simulink model "Quadrotor_Model_CP232"  (R2020a)
settings: Solver=ode3  StartTime=0.0  StopTime=Tf  FixedStep=0.01  RelTol=1e-3  EnableMultiTasking=on
InitFcn:
  | %g = 9.81; % gravity constant m/s^2
  | %m = 0.468; % mass of helicopter kg
  | %l = 0.225; % distance between a rotor and the center of quadcopter (m)
  | %k = 2.98e-6; % lift constant
  | %b = 1.14e-7; % drag constant
  | %I_M = 3.357e-5; % rotational moment of inertia kg.m^2
  | % drag force coefficents
  | %A_x = 0.25; % kg/s
  | %A_y = 0.25;
  | %A_z = 0.25;
  | % inertia matrix
  | %I_xx = 4.856e-3; %kgm^2
  | %I_yy = 4.856e-3;
  | %I_zz = 8.801e-3;
values from neighbouring files (symbols this model uses):
  Fxg = 0.5*scale2    (= 0)    [main_no_wind.m]    (also in main_with_wind.m = 0.005)
  Fyg = 0.5*scale2    (= 0)    [main_no_wind.m]    (also in main_with_wind.m = 0.005)
  g = 9.8    [main_no_wind.m]    (also in main_with_wind.m)
  I = diag([2.3951 2.3951 3.2347])*1e-5    [main_no_wind.m]    (also in main_with_wind.m)
  I_xx = I(1,1)    [main_no_wind.m]    (also in main_with_wind.m)
  I_yy = I(2,2)    [main_no_wind.m]    (also in main_with_wind.m)
  I_zz = I(3,3)    [main_no_wind.m]    (also in main_with_wind.m)
  Kd_eta = [40; 50; 50]    [main_no_wind.m]    (also in main_with_wind.m = [200; 200; 10])
  Kd_zeta = [3; 100; 5]    [main_no_wind.m]    (also in main_with_wind.m = [10; 100; 5])
  kf = 0.005022    [main_no_wind.m]    (also in main_with_wind.m)
  Ki_eta = [0; 0; 0]    [main_no_wind.m]    (also in main_with_wind.m)
  Ki_zeta = [0; 0; 0]    [main_no_wind.m]    (also in main_with_wind.m = [10; 0; 0])
  km = 1.858e-5    (= 1.858e-05)    [main_no_wind.m]    (also in main_with_wind.m)
  Kp_eta = [20; 50; 50]    [main_no_wind.m]    (also in main_with_wind.m = [100; 100; 10])
  Kp_zeta = [2; 1; 1]    [main_no_wind.m]    (also in main_with_wind.m = [50; 50; 10])
  L = 0.032    [main_no_wind.m]    (also in main_with_wind.m)
  m = 0.034    [main_no_wind.m]    (also in main_with_wind.m)
  MMA = [0 kf*L 0 -kf*L;         -kf*L 0 kf*L 0;         km -km km -km]    [main_no_wind.m]    (also in main_with_wind.m)
  scale = 0    [main_no_wind.m]    (also in main_with_wind.m = 0.0001)
  shape = 0    [main_no_wind.m]    (also in main_with_wind.m)
  x_0 = 1    [main_no_wind.m]    (also in main_with_wind.m)
  y_0 = 0    [main_no_wind.m]    (also in main_with_wind.m)
  z_0 = 0    [main_no_wind.m]    (also in main_with_wind.m)
libraries: dspinverses x1
settings Model: Creator=Hamed  LastModifiedBy=Ratnangshu
settings DataIOCC: ReturnWorkspaceOutputs=off
settings OptimizationCC: LifeSpan=inf
settings DebuggingCC: SFUnexpectedBacktrackingDiag=warning  SFNoUnconditionalDefaultTransitionDiag=warning  SFExecutionAtInitializationDiag=none  ArithmeticOperatorsInVariantConditions=warning
settings HardwareCC: ProdBitPerSizeT=32  ProdBitPerPtrDiffT=32  ProdWordSize=32  ProdHWDeviceType=Specified
settings SFSimCC: SimUseLocalCustomCode=off  CustomCodeUndefinedFunction=UseInterfaceOnly
settings RTWCC: RTWUseLocalCustomCode=off
settings CodeAppCC: StateflowObjectComments=on
settings GRTTargetCC: TargetLangStandard=C89/C90 (ANSI)
settings ConfigComp: CovMetricSettings=dw  CovHtmlReporting=on  CovSaveCumulativeToWorkspaceVar=on  CovSaveSingleToWorkspaceVar=on  CovExternalEMLEnable=off

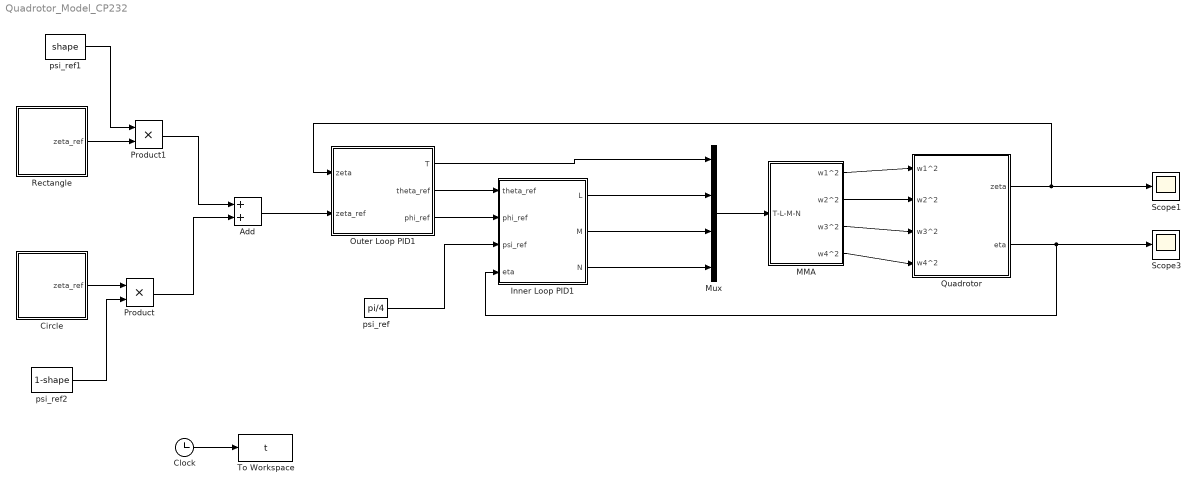
== system Quadrotor_Model_CP232 ==
  Add : Sum
  Circle : Subsystem
  Clock : Clock
  Inner Loop PID1 : Subsystem
  MMA : Subsystem
  Mux : Mux
  Outer Loop PID1 : Subsystem
  Product : Product
  Product1 : Product
  Quadrotor : Subsystem
  Rectangle : Subsystem
  Scope1 : Scope
  Scope3 : Scope
  To Workspace : ToWorkspace  VariableName=t  SampleTime=-1
  psi_ref : Constant  Value=pi/4
  psi_ref1 : Constant  Value=shape
  psi_ref2 : Constant  Value=1-shape
  wires:
  Mux/1 -> MMA/1(T-L-M-N)
  Inner Loop PID1/1(L) -> Mux/2
  Outer Loop PID1/2(theta_ref) -> Inner Loop PID1/1(theta_ref)
  Outer Loop PID1/3(phi_ref) -> Inner Loop PID1/2(phi_ref)
  psi_ref/1 -> Inner Loop PID1/3(psi_ref)
  Outer Loop PID1/1(T) -> Mux/1
  Inner Loop PID1/2(M) -> Mux/3
  Inner Loop PID1/3(N) -> Mux/4
  Quadrotor/1(zeta) -> Outer Loop PID1/1(zeta), Scope1/1
  Quadrotor/2(eta) -> Inner Loop PID1/4(eta), Scope3/1
  MMA/1(w1^2) -> Quadrotor/1(w1^2)
  MMA/2(w2^2) -> Quadrotor/2(w2^2)
  MMA/3(w3^2) -> Quadrotor/3(w3^2)
  MMA/4(w4^2) -> Quadrotor/4(w4^2)
  Add/1 -> Outer Loop PID1/2(zeta_ref)
  Rectangle/1(zeta_ref) -> Product1/2
  Circle/1(zeta_ref) -> Product/1
  Product/1 -> Add/2
  Product1/1 -> Add/1
  psi_ref1/1 -> Product1/1
  psi_ref2/1 -> Product/2
  Clock/1 -> To Workspace/1

== system Quadrotor_Model_CP232/Circle ==
  Clock : Clock
  MATLAB Function : MATLAB Function  TreatAsAtomicUnit=on
  MATLAB Function1 : MATLAB Function  TreatAsAtomicUnit=on
  MATLAB Function2 : MATLAB Function  TreatAsAtomicUnit=on
  Mux : Mux  Inputs=3
  zeta_ref : Outport
  wires:
  Clock/1 -> MATLAB Function2/1(t), MATLAB Function1/1(t), MATLAB Function/1(t)
  MATLAB Function/1(y_ref) -> Mux/2
  MATLAB Function1/1(x_ref) -> Mux/1
  MATLAB Function2/1(z_ref) -> Mux/3
  Mux/1 -> zeta_ref/1

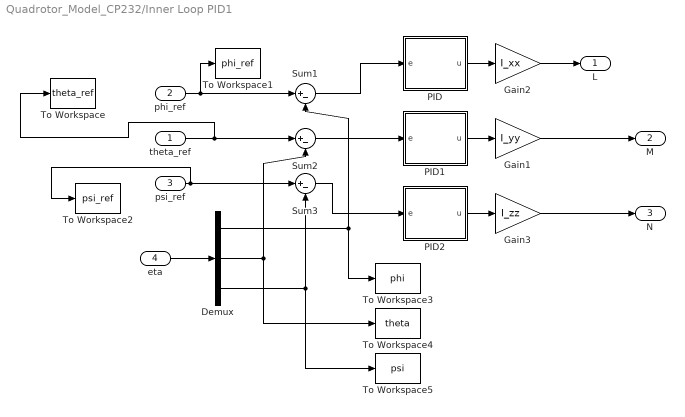
== system Quadrotor_Model_CP232/Inner Loop PID1 ==
  theta_ref : Inport
  phi_ref : Inport  Port=2
  psi_ref : Inport  Port=3
  eta : Inport  Port=4
  Demux : Demux  Outputs=3
  Gain1 : Gain  Gain=I_yy
  Gain2 : Gain  Gain=I_xx
  Gain3 : Gain  Gain=I_zz
  PID : Subsystem
  PID1 : Subsystem
  PID2 : Subsystem
  Sum1 : Sum  Inputs=|+-
  Sum2 : Sum  Inputs=|+-
  Sum3 : Sum  Inputs=|+-
  To Workspace : ToWorkspace  VariableName=theta_ref  SampleTime=-1
  To Workspace1 : ToWorkspace  VariableName=phi_ref  SampleTime=-1
  To Workspace2 : ToWorkspace  VariableName=psi_ref  SampleTime=-1
  To Workspace3 : ToWorkspace  VariableName=phi  SampleTime=-1
  To Workspace4 : ToWorkspace  VariableName=theta  SampleTime=-1
  To Workspace5 : ToWorkspace  VariableName=psi  SampleTime=-1
  L : Outport
  M : Outport  Port=2
  N : Outport  Port=3
  wires:
  PID2/1(u) -> Gain3/1
  PID1/1(u) -> Gain1/1
  PID/1(u) -> Gain2/1
  Gain3/1 -> N/1
  Gain1/1 -> M/1
  Gain2/1 -> L/1
  Demux/2 -> Sum2/2, To Workspace4/1
  Sum2/1 -> PID1/1(e)
  Demux/3 -> Sum3/2, To Workspace5/1
  Sum3/1 -> PID2/1(e)
  Sum1/1 -> PID/1(e)
  theta_ref/1 -> Sum2/1, To Workspace/1
  Demux/1 -> Sum1/2, To Workspace3/1
  phi_ref/1 -> Sum1/1, To Workspace1/1
  psi_ref/1 -> Sum3/1, To Workspace2/1
  eta/1 -> Demux/1

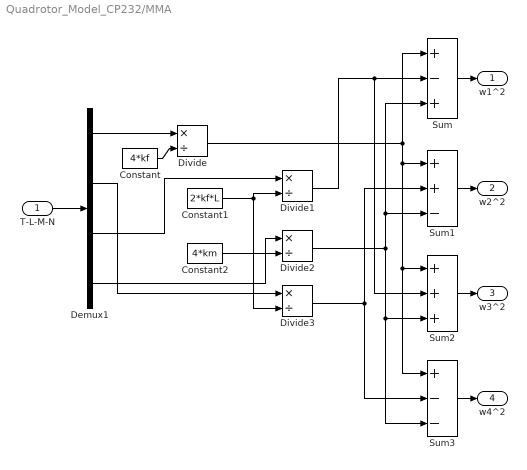
== system Quadrotor_Model_CP232/MMA ==
  T-L-M-N : Inport
  Constant : Constant  Value=4*kf
  Constant1 : Constant  Value=2*kf*L
  Constant2 : Constant  Value=4*km
  Demux1 : Demux
  Divide{,1..3} (4 alike) : Product  Inputs=*/
  Sum : Sum  Inputs=+-+
  Sum1 : Sum  Inputs=++-
  Sum2 : Sum  Inputs=+++
  Sum3 : Sum  Inputs=+--
  w1^2 : Outport
  w2^2 : Outport  Port=2
  w3^2 : Outport  Port=3
  w4^2 : Outport  Port=4
  wires:
  Sum1/1 -> w2^2/1
  T-L-M-N/1 -> Demux1/1
  Sum3/1 -> w4^2/1
  Sum/1 -> w1^2/1
  Demux1/2 -> Divide3/1
  Divide3/1 -> Sum1/2, Sum3/2
  Sum2/1 -> w3^2/1
  Constant/1 -> Divide/2
  Constant2/1 -> Divide2/2
  Demux1/1 -> Divide/1
  Demux1/3 -> Divide1/1
  Demux1/4 -> Divide2/1
  Constant1/1 -> Divide1/2, Divide3/2
  Divide/1 -> Sum/1, Sum3/1, Sum2/1, Sum1/1
  Divide2/1 -> Sum/3, Sum1/3, Sum3/3, Sum2/3
  Divide1/1 -> Sum2/2, Sum/2

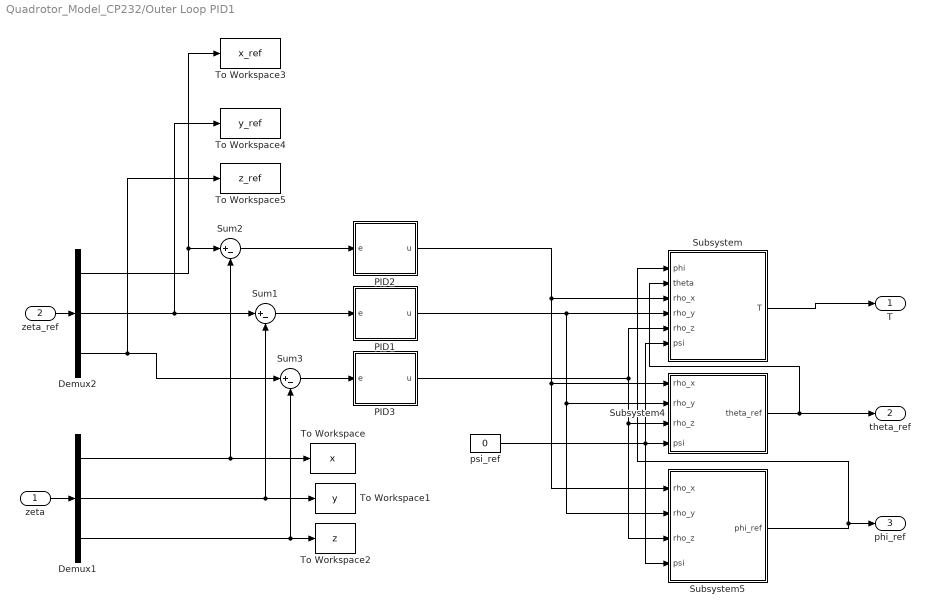
== system Quadrotor_Model_CP232/Outer Loop PID1 ==
  zeta : Inport
  zeta_ref : Inport  Port=2
  Demux1 : Demux  Outputs=3
  Demux2 : Demux  Outputs=3
  PID1 : Subsystem
  PID2 : Subsystem
  PID3 : Subsystem
  Subsystem : Subsystem
  Subsystem4 : Subsystem
  Subsystem5 : Subsystem
  Sum1 : Sum  Inputs=|+-
  Sum2 : Sum  Inputs=|+-
  Sum3 : Sum  Inputs=|+-
  To Workspace : ToWorkspace  VariableName=x  SampleTime=-1
  To Workspace1 : ToWorkspace  VariableName=y  SampleTime=-1
  To Workspace2 : ToWorkspace  VariableName=z  SampleTime=-1
  To Workspace3 : ToWorkspace  VariableName=x_ref  SampleTime=-1
  To Workspace4 : ToWorkspace  VariableName=y_ref  SampleTime=-1
  To Workspace5 : ToWorkspace  VariableName=z_ref  SampleTime=-1
  psi_ref : Constant  Value=0
  T : Outport
  theta_ref : Outport  Port=2
  phi_ref : Outport  Port=3
  wires:
  Sum2/1 -> PID2/1(e)
  Sum3/1 -> PID3/1(e)
  Demux2/3 -> To Workspace5/1, Sum3/1
  Demux2/1 -> To Workspace3/1, Sum2/1
  Demux2/2 -> To Workspace4/1, Sum1/1
  zeta_ref/1 -> Demux2/1
  Demux1/3 -> Sum3/2, To Workspace2/1
  psi_ref/1 -> Subsystem5/4(psi), Subsystem4/4(psi), Subsystem/6(psi)
  Subsystem4/1(theta_ref) -> theta_ref/1, Subsystem/2(theta)
  PID3/1(u) -> Subsystem4/3(rho_z), Subsystem5/3(rho_z), Subsystem/5(rho_z)
  Demux1/2 -> To Workspace1/1, Sum1/2
  Demux1/1 -> Sum2/2, To Workspace/1
  PID1/1(u) -> Subsystem/4(rho_y), Subsystem4/2(rho_y), Subsystem5/2(rho_y)
  zeta/1 -> Demux1/1
  Subsystem/1(T) -> T/1
  Subsystem5/1(phi_ref) -> phi_ref/1, Subsystem/1(phi)
  Sum1/1 -> PID1/1(e)
  PID2/1(u) -> Subsystem/3(rho_x), Subsystem4/1(rho_x), Subsystem5/1(rho_x)

== system Quadrotor_Model_CP232/Quadrotor ==
  w1^2 : Inport
  w2^2 : Inport  Port=2
  w3^2 : Inport  Port=3
  w4^2 : Inport  Port=4
  Rotational Dynamics2 : Subsystem
  Translational Dynamics1 : Subsystem
  zeta : Outport
  eta : Outport  Port=2
  wires:
  w1^2/1 -> Rotational Dynamics2/1(w1^2), Translational Dynamics1/2(w1^2)
  w2^2/1 -> Rotational Dynamics2/2(w2^2), Translational Dynamics1/3(w2^2)
  w3^2/1 -> Rotational Dynamics2/3(w3^2), Translational Dynamics1/4(w3^2)
  Translational Dynamics1/1(zeta) -> zeta/1
  w4^2/1 -> Rotational Dynamics2/4(w4^2), Translational Dynamics1/5(w4^2)
  Rotational Dynamics2/1(eta) -> Translational Dynamics1/1(eta), eta/1

== system Quadrotor_Model_CP232/Rectangle ==
  Clock : Clock
  MATLAB Function : MATLAB Function  TreatAsAtomicUnit=on
  MATLAB Function1 : MATLAB Function  TreatAsAtomicUnit=on
  MATLAB Function2 : MATLAB Function  TreatAsAtomicUnit=on
  Mux : Mux  Inputs=3
  zeta_ref : Outport
  wires:
  MATLAB Function/1(y_ref) -> Mux/2
  MATLAB Function1/1(x_ref) -> Mux/1
  Clock/1 -> MATLAB Function/1(t), MATLAB Function1/1(t), MATLAB Function2/1(t)
  MATLAB Function2/1(z_ref) -> Mux/3
  Mux/1 -> zeta_ref/1

== system Quadrotor_Model_CP232/Inner Loop PID1/PID ==
  e : Inport
  Derivative : Derivative
  Gain : Gain  Gain=Kp_eta(1)
  Gain1 : Gain  Gain=Kd_eta(1)
  Gain2 : Gain  Gain=Ki_eta(1)
  Integrator : Integrator
  Sum2 : Sum  Inputs=+++
  u : Outport
  wires:
  Sum2/1 -> u/1  "u"
  Integrator/1 -> Sum2/2
  Gain2/1 -> Integrator/1
  Gain/1 -> Sum2/1
  Derivative/1 -> Sum2/3
  e/1 -> Gain/1, Gain2/1, Gain1/1
  Gain1/1 -> Derivative/1

== system Quadrotor_Model_CP232/Inner Loop PID1/PID1 ==
  e : Inport
  Derivative : Derivative
  Gain : Gain  Gain=Kp_eta(2)
  Gain1 : Gain  Gain=Kd_eta(2)
  Gain2 : Gain  Gain=Ki_eta(2)
  Integrator : Integrator
  Sum2 : Sum  Inputs=+++
  u : Outport
  wires:
  Gain1/1 -> Derivative/1
  e/1 -> Gain2/1, Gain/1, Gain1/1
  Derivative/1 -> Sum2/3
  Gain/1 -> Sum2/1
  Gain2/1 -> Integrator/1
  Integrator/1 -> Sum2/2
  Sum2/1 -> u/1  "u"

== system Quadrotor_Model_CP232/Inner Loop PID1/PID2 ==
  e : Inport
  Derivative : Derivative
  Gain : Gain  Gain=Kp_eta(3)
  Gain1 : Gain  Gain=Kd_eta(3)
  Gain2 : Gain  Gain=Ki_eta(2)
  Integrator : Integrator
  Sum2 : Sum  Inputs=+++
  u : Outport
  wires:
  Sum2/1 -> u/1  "u"
  Integrator/1 -> Sum2/2
  Gain2/1 -> Integrator/1
  Gain/1 -> Sum2/1
  Derivative/1 -> Sum2/3
  e/1 -> Gain1/1, Gain/1, Gain2/1
  Gain1/1 -> Derivative/1

== system Quadrotor_Model_CP232/Outer Loop PID1/PID1 ==
  e : Inport
  Derivative : Derivative
  Gain : Gain  Gain=Kp_zeta(2)
  Gain1 : Gain  Gain=Kd_zeta(2)
  Gain2 : Gain  Gain=Ki_zeta(2)
  Integrator : Integrator
  Sum2 : Sum  Inputs=+++
  u : Outport
  wires:
  Gain1/1 -> Derivative/1
  e/1 -> Gain2/1, Gain1/1, Gain/1
  Derivative/1 -> Sum2/3
  Gain/1 -> Sum2/1
  Gain2/1 -> Integrator/1
  Integrator/1 -> Sum2/2
  Sum2/1 -> u/1  "u"

== system Quadrotor_Model_CP232/Outer Loop PID1/PID2 ==
  e : Inport
  Derivative : Derivative
  Gain : Gain  Gain=Kp_zeta(1)
  Gain1 : Gain  Gain=Kd_zeta(1)
  Gain2 : Gain  Gain=Ki_zeta(1)
  Integrator : Integrator
  Sum2 : Sum  Inputs=+++
  u : Outport
  wires:
  Sum2/1 -> u/1  "u"
  Integrator/1 -> Sum2/2
  Gain2/1 -> Integrator/1
  Gain/1 -> Sum2/1
  Derivative/1 -> Sum2/3
  e/1 -> Gain1/1, Gain/1, Gain2/1
  Gain1/1 -> Derivative/1

== system Quadrotor_Model_CP232/Outer Loop PID1/PID3 ==
  e : Inport
  Derivative : Derivative
  Gain : Gain  Gain=Kp_zeta(3)
  Gain1 : Gain  Gain=Kd_zeta(3)
  Gain2 : Gain  Gain=Ki_zeta(3)
  Integrator : Integrator
  Sum2 : Sum  Inputs=+++
  u : Outport
  wires:
  Sum2/1 -> u/1  "u"
  Integrator/1 -> Sum2/2
  Gain2/1 -> Integrator/1
  Gain/1 -> Sum2/1
  Derivative/1 -> Sum2/3
  e/1 -> Gain1/1, Gain/1, Gain2/1
  Gain1/1 -> Derivative/1

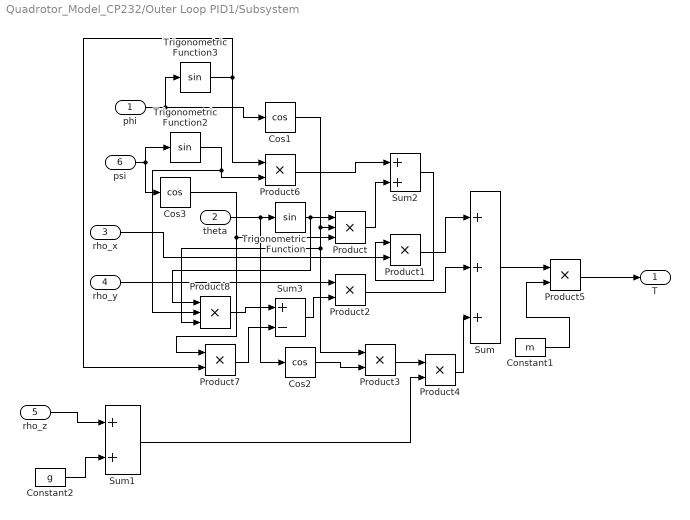
== system Quadrotor_Model_CP232/Outer Loop PID1/Subsystem ==
  phi : Inport
  theta : Inport  Port=2
  rho_x : Inport  Port=3
  rho_y : Inport  Port=4
  rho_z : Inport  Port=5
  psi : Inport  Port=6
  Constant1 : Constant  Value=m
  Constant2 : Constant  Value=g
  Cos1 : Trigonometry  Operator=cos
  Cos2 : Trigonometry  Operator=cos
  Cos3 : Trigonometry  Operator=cos
  Product : Product  Inputs=3  RndMeth=Zero
  Product{1..7} (7 alike) : Product  RndMeth=Zero
  Product8 : Product  Inputs=3  RndMeth=Zero
  Sum : Sum  Inputs=+++
  Sum1 : Sum
  Sum2 : Sum
  Sum3 : Sum  Inputs=+-
  Trigonometric Function : Trigonometry
  Trigonometric Function2 : Trigonometry
  Trigonometric Function3 : Trigonometry
  T : Outport
  wires:
  Product7/1 -> Sum3/2
  Product8/1 -> Sum3/1
  Sum3/1 -> Product2/2
  Sum2/1 -> Product1/1
  Product6/1 -> Sum2/1
  Trigonometric Function3/1 -> Product6/1, Product7/2
  Trigonometric Function2/1 -> Product8/2, Product6/2
  Cos3/1 -> Product/3, Product7/1
  Product/1 -> Sum2/2
  psi/1 -> Cos3/1, Trigonometric Function2/1
  Constant2/1 -> Sum1/2
  rho_z/1 -> Sum1/1
  Sum1/1 -> Product4/2
  Constant1/1 -> Product5/2
  Product5/1 -> T/1
  Sum/1 -> Product5/1
  Product4/1 -> Sum/3
  Product3/1 -> Product4/1
  Cos2/1 -> Product3/2
  Product2/1 -> Sum/2
  rho_y/1 -> Product2/1
  Product1/1 -> Sum/1
  rho_x/1 -> Product1/2
  Cos1/1 -> Product/2, Product3/1, Product8/3
  phi/1 -> Cos1/1, Trigonometric Function3/1
  Trigonometric Function/1 -> Product/1, Product8/1
  theta/1 -> Trigonometric Function/1, Cos2/1

== system Quadrotor_Model_CP232/Outer Loop PID1/Subsystem4 ==
  rho_x : Inport
  rho_y : Inport  Port=2
  rho_z : Inport  Port=3
  psi : Inport  Port=4
  Constant2 : Constant  Value=g
  Divide : Product  Inputs=*/
  Product : Product  RndMeth=Zero
  Product1 : Product  RndMeth=Zero
  Sum : Sum
  Sum1 : Sum
  Trigonometric : Trigonometry  Operator=atan
  Trigonometric1 : Trigonometry  Operator=cos
  Trigonometric2 : Trigonometry
  theta_ref : Outport
  wires:
  Sum1/1 -> Divide/2
  rho_z/1 -> Sum1/1
  Constant2/1 -> Sum1/2
  psi/1 -> Trigonometric2/1, Trigonometric1/1
  Trigonometric/1 -> theta_ref/1
  rho_y/1 -> Product1/1
  rho_x/1 -> Product/1
  Divide/1 -> Trigonometric/1
  Sum/1 -> Divide/1
  Product1/1 -> Sum/2
  Product/1 -> Sum/1
  Trigonometric2/1 -> Product1/2
  Trigonometric1/1 -> Product/2

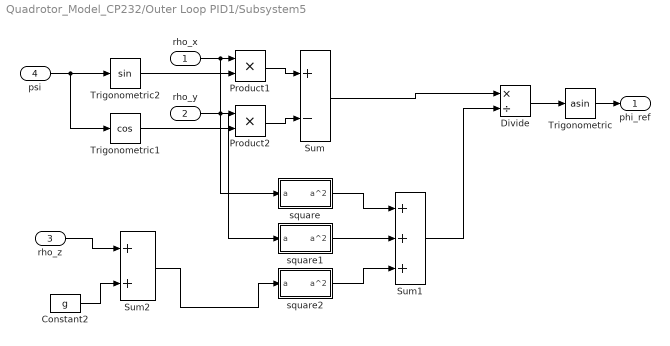
== system Quadrotor_Model_CP232/Outer Loop PID1/Subsystem5 ==
  rho_x : Inport
  rho_y : Inport  Port=2
  rho_z : Inport  Port=3
  psi : Inport  Port=4
  Constant2 : Constant  Value=g
  Divide : Product  Inputs=*/
  Product1 : Product  RndMeth=Zero
  Product2 : Product  RndMeth=Zero
  Sum : Sum  Inputs=+-
  Sum1 : Sum  Inputs=+++
  Sum2 : Sum
  Trigonometric : Trigonometry  Operator=asin
  Trigonometric1 : Trigonometry  Operator=cos
  Trigonometric2 : Trigonometry
  square : Subsystem
  square1 : Subsystem
  square2 : Subsystem
  phi_ref : Outport
  wires:
  Sum2/1 -> square2/1(a)
  rho_z/1 -> Sum2/1
  Constant2/1 -> Sum2/2
  Sum1/1 -> Divide/2
  square2/1(a^2) -> Sum1/3
  square1/1(a^2) -> Sum1/2
  square/1(a^2) -> Sum1/1
  Trigonometric/1 -> phi_ref/1
  rho_y/1 -> Product2/1, square1/1(a)
  rho_x/1 -> Product1/1, square/1(a)
  psi/1 -> Trigonometric1/1, Trigonometric2/1
  Divide/1 -> Trigonometric/1
  Sum/1 -> Divide/1
  Product2/1 -> Sum/2
  Product1/1 -> Sum/1
  Trigonometric1/1 -> Product2/2
  Trigonometric2/1 -> Product1/2

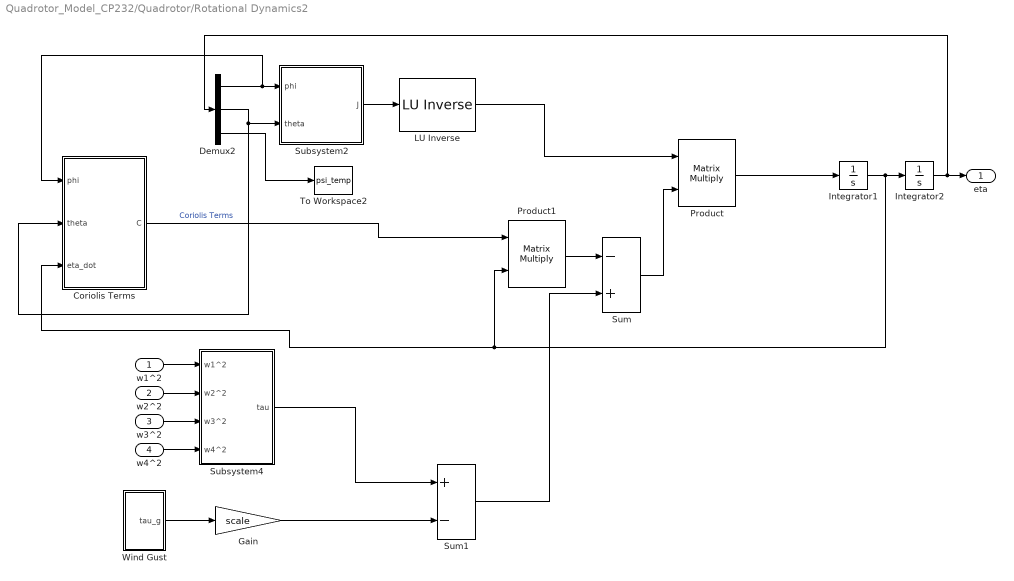
== system Quadrotor_Model_CP232/Quadrotor/Rotational Dynamics2 ==
  w1^2 : Inport
  w2^2 : Inport  Port=2
  w3^2 : Inport  Port=3
  w4^2 : Inport  Port=4
  " LU Inverse" : dspinverses/ LU Inverse
  Coriolis Terms : Subsystem
  Demux2 : Demux  Outputs=3
  Gain : Gain  Gain=scale
  Integrator1 : Integrator  IgnoreLimit=on
  Integrator2 : Integrator  InitialCondition=[0; 0; 0]
  Product : Product  Multiplication=Matrix(*)
  Product1 : Product  Multiplication=Matrix(*)
  Subsystem2 : Subsystem
  Subsystem4 : Subsystem
  Sum : Sum  Inputs=-+
  Sum1 : Sum  Inputs=+-
  To Workspace2 : ToWorkspace  VariableName=psi_temp  SampleTime=-1
  Wind Gust : Subsystem
  eta : Outport
  wires:
  Integrator1/1 -> Product1/2, Coriolis Terms/3(eta_dot), Integrator2/1
  Demux2/1 -> Subsystem2/1(phi), Coriolis Terms/1(phi)
  Sum/1 -> Product/2
  w4^2/1 -> Subsystem4/4(w4^2)
  Demux2/2 -> Subsystem2/2(theta), Coriolis Terms/2(theta)
  w3^2/1 -> Subsystem4/3(w3^2)
  Integrator2/1 -> Demux2/1, eta/1
  w2^2/1 -> Subsystem4/2(w2^2)
  Gain/1 -> Sum1/2
  Coriolis Terms/1(C) -> Product1/1  "Coriolis Terms"
  w1^2/1 -> Subsystem4/1(w1^2)
  Product1/1 -> Sum/1
  Subsystem2/1(J) -> " LU Inverse"/1
  " LU Inverse"/1 -> Product/1
  Wind Gust/1(tau_g) -> Gain/1
  Demux2/3 -> To Workspace2/1
  Product/1 -> Integrator1/1
  Subsystem4/1(tau) -> Sum1/1
  Sum1/1 -> Sum/2

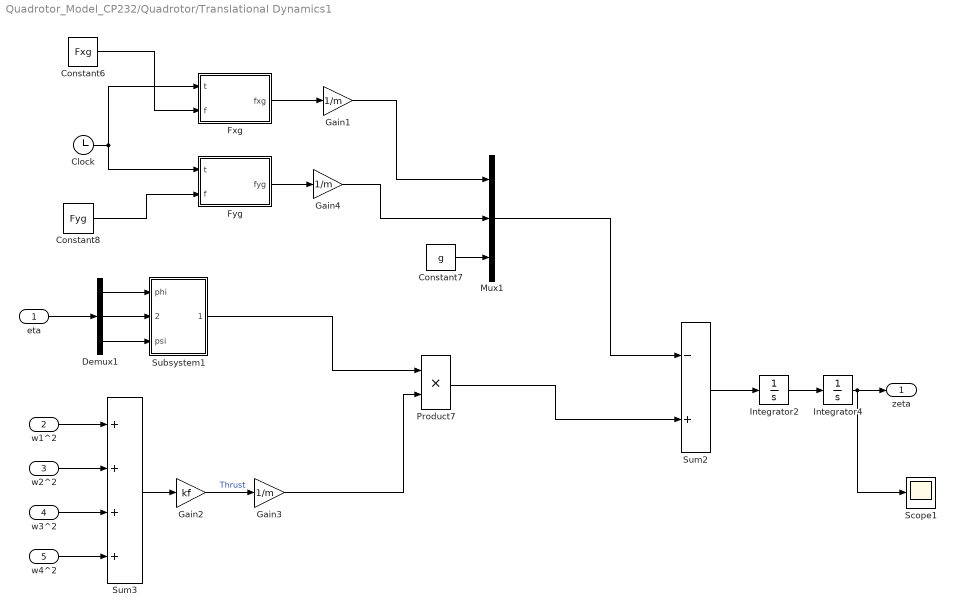
== system Quadrotor_Model_CP232/Quadrotor/Translational Dynamics1 ==
  eta : Inport
  w1^2 : Inport  Port=2
  w2^2 : Inport  Port=3
  w3^2 : Inport  Port=4
  w4^2 : Inport  Port=5
  Clock : Clock
  Constant6 : Constant  Value=Fxg
  Constant7 : Constant  Value=g
  Constant8 : Constant  Value=Fyg
  Demux1 : Demux  Outputs=3
  Fxg : MATLAB Function  TreatAsAtomicUnit=on
  Fyg : MATLAB Function  TreatAsAtomicUnit=on
  Gain1 : Gain  Gain=1/m
  Gain2 : Gain  Gain=kf
  Gain3 : Gain  Gain=1/m
  Gain4 : Gain  Gain=1/m
  Integrator2 : Integrator
  Integrator4 : Integrator  InitialCondition=[x_0; y_0; z_0]
  Mux1 : Mux  Inputs=3
  Product7 : Product
  Scope1 : Scope
  Subsystem1 : Subsystem
  Sum2 : Sum  Inputs=-+
  Sum3 : Sum  Inputs=++++
  zeta : Outport
  wires:
  eta/1 -> Demux1/1
  Demux1/2 -> Subsystem1/2(theta)
  Demux1/3 -> Subsystem1/3(psi)
  Subsystem1/1(Out1) -> Product7/1
  Demux1/1 -> Subsystem1/1(phi)
  Gain2/1 -> Gain3/1  "Thrust"
  Sum3/1 -> Gain2/1
  Constant7/1 -> Mux1/3
  Gain3/1 -> Product7/2
  w4^2/1 -> Sum3/4
  Integrator2/1 -> Integrator4/1
  Mux1/1 -> Sum2/1
  Sum2/1 -> Integrator2/1
  w2^2/1 -> Sum3/2
  w1^2/1 -> Sum3/1
  Integrator4/1 -> Scope1/1, zeta/1
  w3^2/1 -> Sum3/3
  Product7/1 -> Sum2/2
  Fxg/1(fxg) -> Gain1/1
  Fyg/1(fyg) -> Gain4/1
  Clock/1 -> Fxg/1(t), Fyg/1(t)
  Constant6/1 -> Fxg/2(f)
  Constant8/1 -> Fyg/2(f)
  Gain1/1 -> Mux1/1
  Gain4/1 -> Mux1/2

== system Quadrotor_Model_CP232/Outer Loop PID1/Subsystem5/square ==
  a : Inport
  Product : Product  RndMeth=Zero
  a^2 : Outport
  wires:
  Product/1 -> a^2/1
  a/1 -> Product/2, Product/1

== system Quadrotor_Model_CP232/Outer Loop PID1/Subsystem5/square1 ==
  a : Inport
  Product : Product  RndMeth=Zero
  a^2 : Outport
  wires:
  a/1 -> Product/1, Product/2
  Product/1 -> a^2/1

== system Quadrotor_Model_CP232/Outer Loop PID1/Subsystem5/square2 ==
  a : Inport
  Product : Product  RndMeth=Zero
  a^2 : Outport
  wires:
  Product/1 -> a^2/1
  a/1 -> Product/2, Product/1

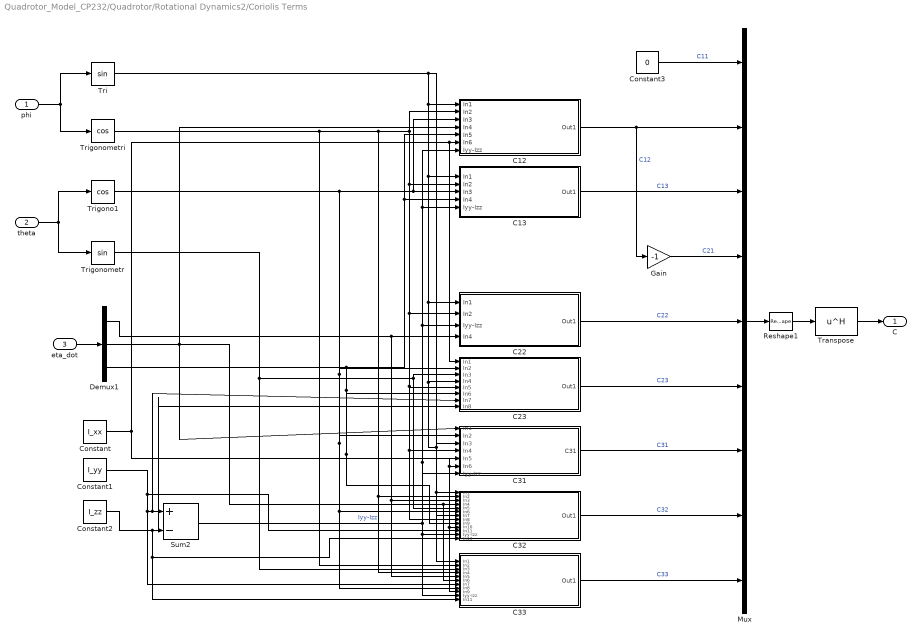
== system Quadrotor_Model_CP232/Quadrotor/Rotational Dynamics2/Coriolis Terms ==
  phi : Inport
  theta : Inport  Port=2
  eta_dot : Inport  Port=3
  C12 : Subsystem
  C13 : Subsystem
  C22 : Subsystem
  C23 : Subsystem
  C31 : Subsystem
  C32 : Subsystem
  C33 : Subsystem
  Constant : Constant  Value=I_xx
  Constant1 : Constant  Value=I_yy
  Constant2 : Constant  Value=I_zz
  Constant3 : Constant  Value=0
  Demux1 : Demux  Outputs=3
  Gain : Gain  Gain=-1
  Mux : Mux  Inputs=9
  Reshape1 : Reshape  OutputDimensionality=Customize  OutputDimensions=[3, 3]
  Sum2 : Sum  Inputs=+-
  Transpose : Math  Operator=hermitian  SignedPower=on
  Tri : Trigonometry
  Trigono1 : Trigonometry  Operator=cos
  Trigonometr : Trigonometry
  Trigonometri : Trigonometry  Operator=cos
  C : Outport
  wires:
  C33/1(Out1) -> Mux/9  "C33"
  Trigonometr/1 -> C33/3(In3), C23/3(In3), C32/5(In5)
  Demux1/1 -> C33/5(In5), C32/3(In3), C22/4(In4)
  C32/1(Out1) -> Mux/8  "C32"
  C22/1(Out1) -> Mux/5  "C22"
  C12/1(Out1) -> Gain/1, Mux/2  "C12"
  Demux1/2 -> C32/4(In4), C33/6(In6), C31/1(In1), C12/4(In4)
  Mux/1 -> Reshape1/1
  Constant2/1 -> C33/11(In11), C32/13(In13), C23/8(In8), Sum2/2
  Trigonometri/1 -> C33/2(In2), C33/4(In4), C32/2(In2), C32/8(In8), C31/4(In4), C23/5(In5), C22/2(In2), C13/2(In2), C12/2(In2)
  Tri/1 -> C33/1(In1), C32/1(In1), C32/7(In7), C31/3(In3), C23/4(In4), C22/1(In1), C13/1(In1), C12/1(In1)
  Constant/1 -> C33/9(In9), C32/10(In10), C31/6(In6), C23/1(In1), C12/6(In6)
  Constant1/1 -> C33/7(In7), C23/7(In7), Sum2/1, C32/11(In11)
  Constant3/1 -> Mux/1  "C11"
  Sum2/1 -> C33/10(Iyy-Izz), C32/12(Iyy-Izz), C12/7(Iyy-Izz), C13/5(Iyy-Izz), C22/3(Iyy-Izz), C31/7(Iyy-Izz)  "Iyy-Izz"
  C31/1(C31) -> Mux/7  "C31"
  Demux1/3 -> C32/9(In9), C31/5(In5), C23/6(In6), C12/5(In5), C13/4(In4)
  Gain/1 -> Mux/4  "C21"
  Trigono1/1 -> C33/8(In8), C32/6(In6), C31/2(In2), C23/2(In2), C12/3(In3), C13/3(In3)
  Reshape1/1 -> Transpose/1
  Transpose/1 -> C/1
  theta/1 -> Trigonometr/1, Trigono1/1
  C23/1(Out1) -> Mux/6  "C23"
  eta_dot/1 -> Demux1/1
  C13/1(Out1) -> Mux/3  "C13"
  phi/1 -> Tri/1, Trigonometri/1

== system Quadrotor_Model_CP232/Quadrotor/Rotational Dynamics2/Subsystem2 ==
  phi : Inport
  theta : Inport  Port=2
  Constant1 : Constant  Value=I
  Matrix Multiply : Product  Inputs=3  Multiplication=Matrix(*)
  Transpose : Math  Operator=hermitian  SignedPower=on
  W : Subsystem
  J : Outport
  wires:
  Matrix Multiply/1 -> J/1
  theta/1 -> W/2(In2)
  W/1(W) -> Transpose/1, Matrix Multiply/3
  Constant1/1 -> Matrix Multiply/2
  Transpose/1 -> Matrix Multiply/1
  phi/1 -> W/1(In1)

== system Quadrotor_Model_CP232/Quadrotor/Rotational Dynamics2/Subsystem4 ==
  w1^2 : Inport
  w2^2 : Inport  Port=2
  w3^2 : Inport  Port=3
  w4^2 : Inport  Port=4
  Constant1 : Constant  Value=MMA
  Matrix Multiply : Product  Multiplication=Matrix(*)
  Mux1 : Mux
  tau : Outport
  wires:
  Matrix Multiply/1 -> tau/1
  Constant1/1 -> Matrix Multiply/1
  Mux1/1 -> Matrix Multiply/2  "tau"
  w3^2/1 -> Mux1/3
  w2^2/1 -> Mux1/2
  w1^2/1 -> Mux1/1
  w4^2/1 -> Mux1/4

== system Quadrotor_Model_CP232/Quadrotor/Rotational Dynamics2/Wind Gust ==
  Clock : Clock
  Fxg : MATLAB Function  TreatAsAtomicUnit=on
  Fyg : MATLAB Function  TreatAsAtomicUnit=on
  Fyg1 : MATLAB Function  TreatAsAtomicUnit=on
  Mux1 : Mux  Inputs=3
  tau_g : Outport
  wires:
  Mux1/1 -> tau_g/1  "tau_g"
  Clock/1 -> Fyg1/1(t), Fyg/1(t), Fxg/1(t)
  Fyg/1(tau_g_2) -> Mux1/2
  Fyg1/1(tau_g_3) -> Mux1/3
  Fxg/1(tau_g_1) -> Mux1/1

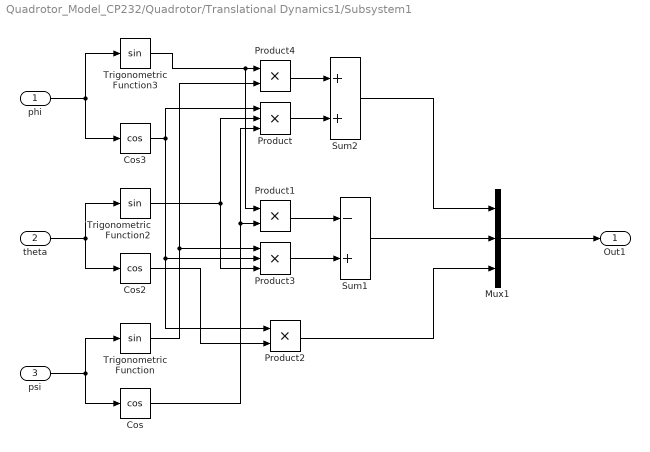
== system Quadrotor_Model_CP232/Quadrotor/Translational Dynamics1/Subsystem1 ==
  phi : Inport
  theta : Inport  Port=2
  psi : Inport  Port=3
  Cos : Trigonometry  Operator=cos
  Cos2 : Trigonometry  Operator=cos
  Cos3 : Trigonometry  Operator=cos
  Mux1 : Mux  Inputs=3
  Product : Product  Inputs=3
  Product1 : Product
  Product2 : Product
  Product3 : Product  Inputs=3
  Product4 : Product
  Sum1 : Sum  Inputs=-+
  Sum2 : Sum
  Trigonometric Function : Trigonometry
  Trigonometric Function2 : Trigonometry
  Trigonometric Function3 : Trigonometry
  Out1 : Outport
  wires:
  Product2/1 -> Mux1/3
  Sum1/1 -> Mux1/2
  Sum2/1 -> Mux1/1
  Cos2/1 -> Product2/2
  Product3/1 -> Sum1/2
  Product1/1 -> Sum1/1
  Product/1 -> Sum2/2
  Product4/1 -> Sum2/1
  Trigonometric Function2/1 -> Product/2, Product3/3
  Cos3/1 -> Product/1, Product3/2, Product2/1
  Cos/1 -> Product/3, Product1/2
  Trigonometric Function3/1 -> Product4/1, Product1/1
  Trigonometric Function/1 -> Product4/2, Product3/1
  phi/1 -> Trigonometric Function3/1, Cos3/1
  theta/1 -> Trigonometric Function2/1, Cos2/1
  psi/1 -> Trigonometric Function/1, Cos/1
  Mux1/1 -> Out1/1

== system Quadrotor_Model_CP232/Quadrotor/Rotational Dynamics2/Coriolis Terms/C12 ==
  In1 : Inport
  In2 : Inport  Port=2
  In3 : Inport  Port=3
  In4 : Inport  Port=4
  In5 : Inport  Port=5
  In6 : Inport  Port=6
  Iyy-Izz : Inport  Port=7
  Gain : Gain  Gain=-1
  Product : Product  Inputs=3
  Product1 : Product  Inputs=4
  Product2 : Product
  Product3 : Product  Inputs=5
  Product4 : Product  Inputs=3
  Sum3 : Sum
  Sum5 : Sum  Inputs=+++
  Out1 : Outport
  wires:
  In2/1 -> Product/2, Product3/4, Product3/3
  Product2/1 -> Sum5/1
  Product/1 -> Sum3/1
  In1/1 -> Product1/2, Product1/3, Product/3
  Iyy-Izz/1 -> Gain/1, Product2/2
  In5/1 -> Product3/2, Product4/2, Product1/1
  In3/1 -> Product3/5, Product4/3, Product1/4
  Product4/1 -> Sum5/3
  Gain/1 -> Product3/1
  Sum5/1 -> Out1/1
  Product1/1 -> Sum3/2
  Product3/1 -> Sum5/2
  Sum3/1 -> Product2/1  "Ixx-Iyy"
  In4/1 -> Product/1
  In6/1 -> Product4/1

== system Quadrotor_Model_CP232/Quadrotor/Rotational Dynamics2/Coriolis Terms/C13 ==
  In1 : Inport
  In2 : Inport  Port=2
  In3 : Inport  Port=3
  In4 : Inport  Port=4
  Iyy-Izz : Inport  Port=5
  Gain1 : Gain  Gain=-1
  Product1 : Product  Inputs=6
  Out1 : Outport
  wires:
  Iyy-Izz/1 -> Gain1/1
  Product1/1 -> Out1/1
  In3/1 -> Product1/6, Product1/5
  In4/1 -> Product1/2
  In2/1 -> Product1/4
  Gain1/1 -> Product1/1
  In1/1 -> Product1/3

== system Quadrotor_Model_CP232/Quadrotor/Rotational Dynamics2/Coriolis Terms/C22 ==
  In1 : Inport
  In2 : Inport  Port=2
  Iyy-Izz : Inport  Port=3
  In4 : Inport  Port=4
  Gain1 : Gain  Gain=-1
  Product1 : Product  Inputs=4
  Out1 : Outport
  wires:
  Gain1/1 -> Product1/1
  Product1/1 -> Out1/1
  In2/1 -> Product1/4
  Iyy-Izz/1 -> Gain1/1
  In4/1 -> Product1/2
  In1/1 -> Product1/3

== system Quadrotor_Model_CP232/Quadrotor/Rotational Dynamics2/Coriolis Terms/C23 ==
  In1 : Inport
  In2 : Inport  Port=2
  In3 : Inport  Port=3
  In4 : Inport  Port=4
  In5 : Inport  Port=5
  In6 : Inport  Port=6
  In7 : Inport  Port=7
  In8 : Inport  Port=8
  Product1 : Product
  Product2 : Product  Inputs=3
  Product3 : Product  Inputs=4
  Product4 : Product  Inputs=4
  Sum5 : Sum  Inputs=-++
  Out1 : Outport
  wires:
  In1/1 -> Product1/1
  Product4/1 -> Sum5/3
  Product2/1 -> Product3/2, Product4/2, Product1/2
  In3/1 -> Product2/2
  Product1/1 -> Sum5/1
  In4/1 -> Product3/4, Product3/3
  Product3/1 -> Sum5/2
  In5/1 -> Product4/4, Product4/3
  In8/1 -> Product4/1
  Sum5/1 -> Out1/1
  In6/1 -> Product2/3
  In7/1 -> Product3/1
  In2/1 -> Product2/1

== system Quadrotor_Model_CP232/Quadrotor/Rotational Dynamics2/Coriolis Terms/C31 ==
  In1 : Inport
  In2 : Inport  Port=2
  In3 : Inport  Port=3
  In4 : Inport  Port=4
  In5 : Inport  Port=5
  In6 : Inport  Port=6
  Iyy-Izz : Inport  Port=7
  Product1 : Product  Inputs=6
  Product2 : Product  Inputs=3
  Sum5 : Sum  Inputs=+-
  C31 : Outport
  wires:
  Sum5/1 -> C31/1  "C31"
  Product2/1 -> Sum5/2
  In2/1 -> Product2/3, Product1/4, Product1/3
  Iyy-Izz/1 -> Product1/1
  Product1/1 -> Sum5/1
  In1/1 -> Product2/2
  In4/1 -> Product1/6
  In5/1 -> Product1/2
  In6/1 -> Product2/1
  In3/1 -> Product1/5

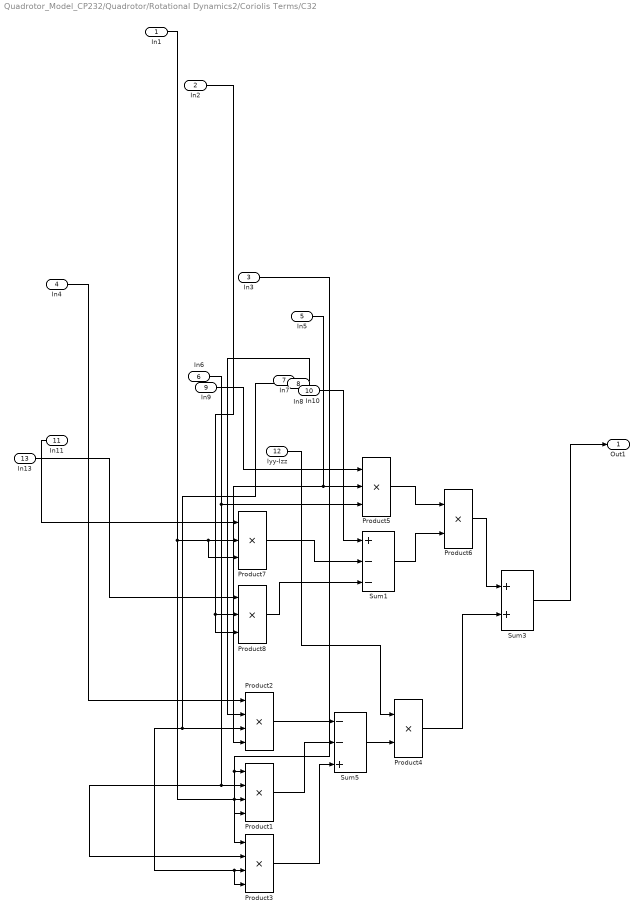
== system Quadrotor_Model_CP232/Quadrotor/Rotational Dynamics2/Coriolis Terms/C32 ==
  In1 : Inport
  In2 : Inport  Port=2
  In3 : Inport  Port=3
  In4 : Inport  Port=4
  In5 : Inport  Port=5
  In6 : Inport  Port=6
  In7 : Inport  Port=7
  In8 : Inport  Port=8
  In9 : Inport  Port=9
  In10 : Inport  Port=10
  In11 : Inport  Port=11
  Iyy-Izz : Inport  Port=12
  In13 : Inport  Port=13
  Product1 : Product  Inputs=4
  Product2 : Product  Inputs=4
  Product3 : Product  Inputs=4
  Product4 : Product
  Product5 : Product  Inputs=3
  Product6 : Product
  Product7 : Product  Inputs=3
  Product8 : Product  Inputs=3
  Sum1 : Sum  Inputs=+--
  Sum3 : Sum
  Sum5 : Sum  Inputs=--+
  Out1 : Outport
  wires:
  In6/1 -> Product5/3, Product3/2, Product1/2
  Product3/1 -> Sum5/3
  In8/1 -> Product3/4, Product3/3, Product2/3
  Product2/1 -> Sum5/1
  Sum5/1 -> Product4/2
  In10/1 -> Sum1/1
  Product5/1 -> Product6/1
  In2/1 -> Product8/3, Product8/2
  Sum3/1 -> Out1/1
  In1/1 -> Product1/4, Product1/3, Product7/3, Product7/2
  Product4/1 -> Sum3/2
  In5/1 -> Product2/4, Product5/2
  Product8/1 -> Sum1/3
  Product6/1 -> Sum3/1
  In7/1 -> Product2/2
  Sum1/1 -> Product6/2
  Product1/1 -> Sum5/2
  Product7/1 -> Sum1/2
  In3/1 -> Product3/1, Product1/1
  In11/1 -> Product7/1
  In9/1 -> Product5/1
  Iyy-Izz/1 -> Product4/1
  In4/1 -> Product2/1
  In13/1 -> Product8/1

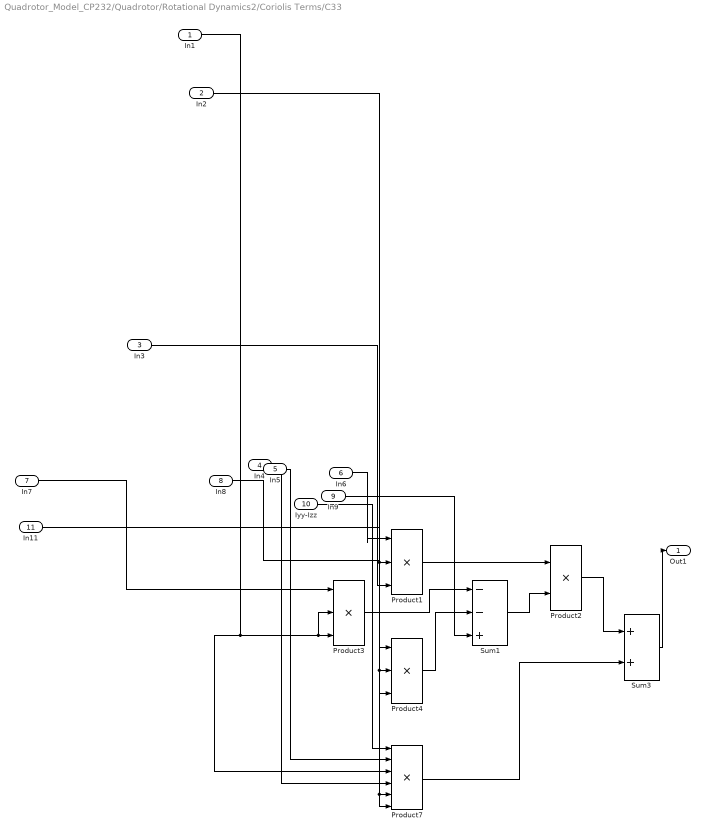
== system Quadrotor_Model_CP232/Quadrotor/Rotational Dynamics2/Coriolis Terms/C33 ==
  In1 : Inport
  In2 : Inport  Port=2
  In3 : Inport  Port=3
  In4 : Inport  Port=4
  In5 : Inport  Port=5
  In6 : Inport  Port=6
  In7 : Inport  Port=7
  In8 : Inport  Port=8
  In9 : Inport  Port=9
  Iyy-Izz : Inport  Port=10
  In11 : Inport  Port=11
  Product1 : Product  Inputs=3
  Product2 : Product
  Product3 : Product  Inputs=3
  Product4 : Product  Inputs=3
  Product7 : Product  Inputs=6
  Sum1 : Sum  Inputs=--+
  Sum3 : Sum
  Out1 : Outport
  wires:
  Product2/1 -> Sum3/1
  In8/1 -> Product1/2, Product7/6, Product7/5
  Product4/1 -> Sum1/2
  In2/1 -> Product4/3, Product4/2
  Product7/1 -> Sum3/2
  In1/1 -> Product7/3, Product3/3, Product3/2
  Sum1/1 -> Product2/2
  Product3/1 -> Sum1/1
  In5/1 -> Product7/2
  Product1/1 -> Product2/1
  In9/1 -> Sum1/3
  In6/1 -> Product1/1
  Iyy-Izz/1 -> Product7/1
  In4/1 -> Product7/4
  Sum3/1 -> Out1/1
  In7/1 -> Product3/1
  In3/1 -> Product1/3
  In11/1 -> Product4/1

== system Quadrotor_Model_CP232/Quadrotor/Rotational Dynamics2/Subsystem2/W ==
  In1 : Inport
  In2 : Inport  Port=2
  Constant1 : Constant
  Constant3 : Constant  Value=0
  Gain : Gain  Gain=-1
  Gain1 : Gain  Gain=-1
  Mux1 : Mux  Inputs=9
  Product : Product
  Product1 : Product
  Reshape2 : Reshape  OutputDimensionality=Customize  OutputDimensions=[3, 3]
  Trigonometri1 : Trigonometry  Operator=cos
  Trigonometri2 : Trigonometry  Operator=cos
  Trigonometric Function1 : Trigonometry
  Trigonometric Function2 : Trigonometry
  W : Outport
  wires:
  Reshape2/1 -> W/1
  Gain/1 -> Mux1/3
  Product/1 -> Mux1/6
  Mux1/1 -> Reshape2/1
  Trigonometric Function1/1 -> Gain/1
  In1/1 -> Trigonometric Function1/1, Trigonometri2/1
  Trigonometri2/1 -> Product1/1, Product/1
  Constant3/1 -> Mux1/2, Mux1/4, Mux1/7
  Trigonometric Function2/1 -> Product/2, Gain1/1
  In2/1 -> Trigonometri1/1, Trigonometric Function2/1
  Product1/1 -> Mux1/9
  Constant1/1 -> Mux1/1
  Gain1/1 -> Mux1/8
  Trigonometri1/1 -> Mux1/5, Product1/2

== matlab function Quadrotor_Model_CP232/Circle/MATLAB Function ==
  data: t input; y_ref output
function y_ref = fcn(t)
%#codegen
if t < 10
    y_ref = 0; % Take Off
elseif t>=10 && t<50
    th = (t-10)/40*2*pi; % 0 -> 2\pi
    y_ref = sin(th);
elseif t>=50 && t<60
    y_ref = 0; % Landing
else 
    y_ref = 0;
end

== matlab function Quadrotor_Model_CP232/Rectangle/MATLAB Function ==
  data: t input; y_ref output
function y_ref = fcn(t)
%#codegen
if t < 10
    y_ref = 2; % Take Off
elseif t>=10 && t<20
    y_ref = 2; % 2
elseif t>=20 && t<30
    y_ref = 4 - t/10; % 2 -> 1
elseif t>=30 && t<40
    y_ref = 1; % 1 
elseif t>=40 && t<50
    y_ref = -3 + t/10; % 1 -> 2
elseif t>=50 && t<60
    y_ref = 2; % Landing
else 
    y_ref = 2;
end

== matlab function Quadrotor_Model_CP232/Rectangle/MATLAB Function1 ==
  data: t input; x_ref output
function x_ref = fcn(t)
%#codegen
if t < 10
    x_ref = 2; % Take Off
elseif t>=10 && t<20
    x_ref = 3 - t/10; % 2 -> 1
elseif t>=20 && t<30
    x_ref = 1; % 1
elseif t>=30 && t<40
    x_ref = -2 + t/10; % 1 -> 2
elseif t>=40 && t<50
    x_ref = 2; % 2
elseif t>=50 && t<60
    x_ref = 2; % Landing
else 
    x_ref = 2;
end

== matlab function Quadrotor_Model_CP232/Circle/MATLAB Function1 ==
  data: t input; x_ref output
function x_ref = fcn(t)
%#codegen
if t < 10
    x_ref = 1; % Take Off
elseif t>=10 && t<50
    th = (t-10)/40*2*pi; % 0 -> 2\pi
    x_ref = cos(th); 
elseif t>=50 && t<60
    x_ref = 1; % Landing
else 
    x_ref = 1;
end

== matlab function Quadrotor_Model_CP232/Circle/MATLAB Function2 ==
  data: t input; z_ref output
function z_ref = fcn(t)
%#codegen
if t < 10
    z_ref = t/10; % Take Off
elseif t>=10 && t<50
    z_ref = 1; % Altitude Hold
elseif t>=50 && t<60
    z_ref = 6 - t/10; % Landing
else 
    z_ref = 0;
end

== matlab function Quadrotor_Model_CP232/Quadrotor/Translational Dynamics1/Fyg ==
  data: t input; fyg output; f input
function fyg = fcn(t,f)
%#codegen
if t < 2
    fyg = 0; % Take Off
elseif t>=2 && t<58
    fyg = f; 
elseif t>=58 && t<60
    fyg = 0; % Landing
else 
    fyg = 0;
end

== matlab function Quadrotor_Model_CP232/Quadrotor/Translational Dynamics1/Fxg ==
  data: t input; fxg output; f input
function fxg = fcn(t,f)
%#codegen
if t < 2
    fxg = 0; % Take Off
elseif t>=2 && t<58
    fxg = f; 
elseif t>=58 && t<60
    fxg = 0; % Landing
else 
    fxg = 0;
end

== matlab function Quadrotor_Model_CP232/Quadrotor/Rotational Dynamics2/Wind Gust/Fxg ==
  data: t input; tau_g_1 output
function tau_g_1 = fcn(t)
%#codegen
if t < 2
    tau_g_1 = 0; % Take Off
elseif t>=2 && t<58
    tau_g_1 = cos(t); 
elseif t>=58 && t<60
    tau_g_1 = 0; % Landing
else 
    tau_g_1 = 0;
end

== matlab function Quadrotor_Model_CP232/Quadrotor/Rotational Dynamics2/Wind Gust/Fyg ==
  data: t input; tau_g_2 output
function tau_g_2 = fcn(t)
%#codegen
if t < 2
    tau_g_2 = 0; % Take Off
elseif t>=2 && t<58
    tau_g_2 = sin(t); 
elseif t>=58 && t<60
    tau_g_2 = 0; % Landing
else 
    tau_g_2 = 0;
end

== matlab function Quadrotor_Model_CP232/Rectangle/MATLAB Function2 ==
  data: t input; z_ref output
function z_ref = fcn(t)
%#codegen
if t < 10
    z_ref = t/10; % Take Off
elseif t>=10 && t<50
    z_ref = 1; % Altitude Hold
elseif t>=50 && t<60
    z_ref = 6 - t/10; % Landing
else 
    z_ref = 0;
end

== matlab function Quadrotor_Model_CP232/Quadrotor/Rotational Dynamics2/Wind Gust/Fyg1 ==
  data: t input; tau_g_3 output
function tau_g_3 = fcn(t)
%#codegen
if t < 2
    tau_g_3 = 0; % Take Off
elseif t>=2 && t<58
    tau_g_3 = 2*sin(t); 
elseif t>=58 && t<60
    tau_g_3 = 0; % Landing
else 
    tau_g_3 = 0;
end
